simulink model "EHRTC_transfer_functions"  (R2018b)
settings: Solver=VariableStepAuto  StartTime=0.0  StopTime=12000  RelTol=1e-3
undefined symbols (not defined in the file): kc, kE, kp, Tc, Tp
settings Model: Creator=bogda  LastModifiedBy=bogda

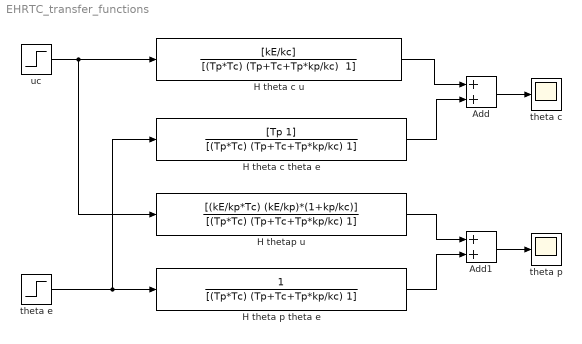
== system EHRTC_transfer_functions ==
  Add : Sum
  Add1 : Sum
  H theta c theta e : TransferFcn  Numerator=[Tp 1]  Denominator=[(Tp*Tc) (Tp+Tc+Tp*kp/kc) 1]
  H theta c u : TransferFcn  Numerator=[kE/kc]  Denominator="[(Tp*Tc) (Tp+Tc+Tp*kp/kc)  1]"
  H theta p theta e : TransferFcn  Denominator=[(Tp*Tc) (Tp+Tc+Tp*kp/kc) 1]
  H thetap u : TransferFcn  Numerator=[(kE/kp*Tc) (kE/kp)*(1+kp/kc)]  Denominator=[(Tp*Tc) (Tp+Tc+Tp*kp/kc) 1]
  theta c : Scope
  theta e : Step  Time=5000  After=-10  SampleTime=0
  theta p : Scope
  uc : Step  Time=0  After=2.5  SampleTime=0
  wires:
  uc/1 -> H thetap u/1, H theta c u/1
  theta e/1 -> H theta p theta e/1, H theta c theta e/1
  H theta c theta e/1 -> Add/2
  H theta c u/1 -> Add/1
  Add/1 -> theta c/1
  H thetap u/1 -> Add1/1
  H theta p theta e/1 -> Add1/2
  Add1/1 -> theta p/1
